simulink model "drive_closed_loop_system"  (R2023b)
settings: Solver=FixedStepDiscrete  StartTime=0.0  StopTime=0.1  FixedStep=Ts  RelTol=1e-3
model workspace (MATLAB code in the model file):
  | % Top-level execution parameter
  | % Placeholder value for structural closed-loop execution only.
  | 
  | Ts = 1e-6;      % top-level discrete step [s]
  | 
  | % Neutral default operating point for Phase-4 behavioural baseline
  | i_d_ref_default = 0;
  | i_q_ref_default = 10;
  | omega_e_default = 300;
  | 
  | % Current step response setup
  | i_q_ref_step_t = 0.02;
  | i_q_ref_step_init = i_q_ref_default;
  | i_q_ref_step_final = i_q_ref_default;
  | 
  | % Load disturbance setup
  | omega_e_step_t = 0.02;
  | omega_e_init = omega_e_default;
  | omega_e_step_final = omega_e_default;
undefined symbols (not defined in the file): DiscIntNeverNeededParam
libraries: sps_lib x1
settings Model: Creator=hwma  LastModifiedBy=hwma

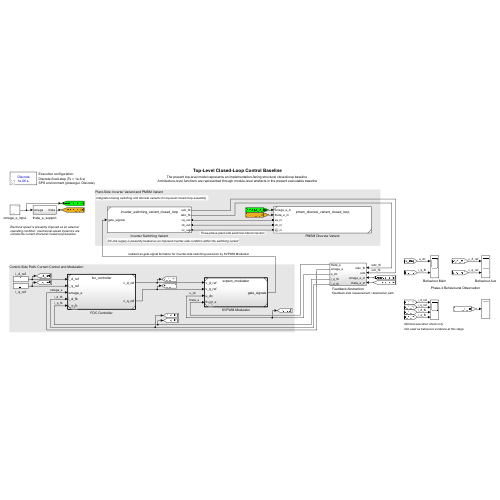
[thumbnail: Simulink's stored preview of the top-level diagram]
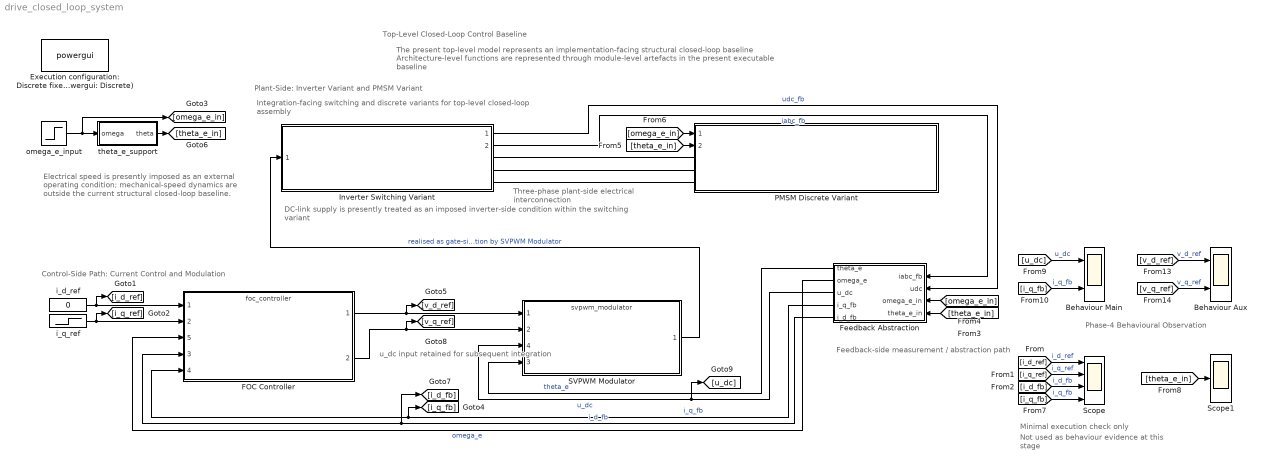
== system drive_closed_loop_system ==
  note: Phase-4 Behavioural Observation
  note: Minimal execution check only
  note: DC-link supply is presently treated as an imposed inverter-side condition within the switching variant
  note: Electrical speed is presently imposed as an external operating condition; mechanical-speed dynamics are outside the current structural closed-loop baseline.
  note: Three-phase plant-side electrical interconnection
  note: Feedback-side measurement / abstraction path
  note: Integration-facing switching and discrete variants for top-level closed-loop assembly
  note: Control-Side Path: Current Control and Modulation
  note: u_dc input retained for subsequent integration
  note: The present top-level model represents an implementation-facing structural closed-loop baseline
      | Architecture-level functions are represented through module-level artefacts in the present executable baseline
  note: Top-Level Closed-Loop Control Baseline
  note: Plant-Side: Inverter Variant and PMSM Variant
  note: Not used as behaviour evidence at this stage
  Behaviour Aux : Scope  NumInputPorts=2
  Behaviour Main : Scope  NumInputPorts=2
  Execution configuration: Discrete fixed-step (Ts = 1e-6 s) SPS environment (powergui: Discrete) : sps_lib/powergui  Priority=1  SimulationMode=Discrete  SampleTime=Ts  frequency=60  Iterations=50  frequencyindice=0  Pbase=100e6  ErrMax=1e-4  UnitsV=kV  UnitsW=MW  buscounter=0  FunctionMessages=off  echomessages=off  EnableUseOfTLC=off  CurrentSourceSwitches=off  DisableSnubberDevices=off  DisableRonSwitches=off  DisableVfSwitches=off  DisplayEquations=off  AutomaticDiscreteSolvers=off  SolverType=Tustin/Backward Euler (TBE)  Interpol=off  ExternalGateDelay=off  methode=off  Ts=100  x0status=blocks  SPID=on  SwTol=0  HookPort=off  NonlinearTolerance=1e-4  nMaxIteration=100  ContinueOnMaxIteration=off  RestoreLinks=warning  ResistiveCurrentMeasurement=off  Frange=[0:2:500]  Ylog=off  Xlog=on  ShowGrid=off  save=off  variable=ZData  structure=0  ZoomFFT=off  StartTime=0.0  cycles=1  DisplayStyle=1  fundamental=60  FreqAxis=off  MaxFrequency=1000  frequencyindicesteady=1  RmsSteady=1  display=off
  FOC Controller : ModelReference  ModelNameDialog=foc_controller.slx  SimulationMode=Normal  ModelReferenceVersion=1.26
      settings: PortSchema="{\"entries\":[{\"content\":{\"sides\":[{\"content\":{\"connectorIds\":[\"In1\",\"In2\",\"In5\",\"In3\",\"In4\"]},\"type\":\"ConnectorPlacement.EquallySpacedRectSide\",\"uuid\":\"ef112b4b-a133-4498-b633-78f8f1506d01\"},{\"content\":{\"connectorIds\":[\"Out1\",\"Out2\"],\"side\":\"RIGHT\"},\"type\":\"ConnectorPlacement.EquallySpacedRectSide\",\"uuid\":\"9847a18b-aaef-4243-aa5c-65f99a7910c1\"},{\"content\":{\"side\":\"TOP\"},\"type\":\"ConnectorPlacement.EquallySpacedRectSide\",\"uuid\":\"77b91c6a-a91c-4edb-91a8-4515c999bc11\"}]},\"type\":\"ConnectorPlacement.EquallySpacedConnector\",\"uuid\":\"240ede47-394a-4747-9d30-c9f3a7878d8f\"}],\"packageUris\":[\"http://schema.mathworks.com/mf0/Connector/R2020b\"],\"version\":\"1.0\"}"
  Feedback Abstraction : Subsystem
  Inverter Switching Variant : Subsystem  ReferencedSubsystem=inverter_switching_variant_closed_loop
  PMSM Discrete Variant : Subsystem  ReferencedSubsystem=pmsm_discrete_variant_closed_loop  Rs=0.05  Ld=2e-3  Lq=2e-3  lambda_f=0.1
  SVPWM Modulator : ModelReference  ModelNameDialog=svpwm_modulator.slx  SimulationMode=Normal  ModelReferenceVersion=1.34
      settings: PortSchema="{\"entries\":[{\"content\":{\"sides\":[{\"content\":{\"connectorIds\":[\"In1\",\"In2\",\"In4\",\"In3\"]},\"type\":\"ConnectorPlacement.EquallySpacedRectSide\",\"uuid\":\"0e0645a3-2a27-4c15-9a47-960d3777f31f\"},{\"content\":{\"connectorIds\":[\"Out1\"],\"side\":\"RIGHT\"},\"type\":\"ConnectorPlacement.EquallySpacedRectSide\",\"uuid\":\"17890dc1-ee5f-46a3-bfa4-af9c9726f2d2\"},{\"content\":{\"side\":\"TOP\"},\"type\":\"ConnectorPlacement.EquallySpacedRectSide\",\"uuid\":\"20a4fc6c-c015-4803-8581-584a4f0c357e\"}]},\"type\":\"ConnectorPlacement.EquallySpacedConnector\",\"uuid\":\"32cc6c3a-ba2d-4e41-b4c2-e07b22b54d61\"}],\"packageUris\":[\"http://schema.mathworks.com/mf0/Connector/R2020b\"],\"version\":\"1.0\"}"
  Scope : Scope  NumInputPorts=4
  Scope1 : Scope
  i_d_ref : Constant  Value=0  SampleTime=Ts
  i_q_ref : Step  Time=i_q_ref_step_t  Before=i_q_ref_step_init  After=i_q_ref_step_final  SampleTime=Ts
  omega_e_input : Step  Time=omega_e_step_t  Before=omega_e_init  After=omega_e_step_final  SampleTime=Ts
  theta_e_support : Subsystem
  wires:
  i_d_ref/1 -> FOC Controller/1, [i_d_ref]
  i_q_ref/1 -> [i_q_ref], FOC Controller/2
  FOC Controller/1 -> [v_d_ref], SVPWM Modulator/1
  FOC Controller/2 -> [v_q_ref], SVPWM Modulator/2
  SVPWM Modulator/1 -> Inverter Switching Variant/1  "realised as gate-signal formation for inverter-side switching execution by SVPWM Modulator"
  Inverter Switching Variant/1 -> Feedback Abstraction/2(udc)  "udc_fb"
  Inverter Switching Variant/2 -> Feedback Abstraction/1(iabc_fb)  "iabc_fb"
  Feedback Abstraction/5(i_d_fb) -> [i_d_fb], FOC Controller/3  "i_d_fb"
  Feedback Abstraction/4(i_q_fb) -> [i_q_fb], FOC Controller/4  "i_q_fb"
  Feedback Abstraction/3(u_dc) -> [u_dc], SVPWM Modulator/4  "u_dc"
  [omega_e_in] -> Feedback Abstraction/3(omega_e_in)
  omega_e_input/1 -> theta_e_support/1(omega), [omega_e_in]
  [theta_e_in] -> Feedback Abstraction/4(theta_e_in)
  [theta_e_in] -> PMSM Discrete Variant/2
  [omega_e_in] -> PMSM Discrete Variant/1
  Feedback Abstraction/1(theta_e) -> SVPWM Modulator/3  "theta_e"
  Feedback Abstraction/2(omega_e) -> FOC Controller/5  "omega_e"
  theta_e_support/1(theta) -> [theta_e_in]
  [i_d_ref] -> Scope/1  "i_d_ref"
  [i_q_ref] -> Scope/2  "i_q_ref"
  [i_d_fb] -> Scope/3  "i_d_fb"
  [i_q_fb] -> Scope/4  "i_q_fb"
  [theta_e_in] -> Scope1/1
  [u_dc] -> Behaviour Main/1  "u_dc"
  [i_q_fb] -> Behaviour Main/2  "i_q_fb"
  [v_q_ref] -> Behaviour Aux/2  "v_q_ref"
  [v_d_ref] -> Behaviour Aux/1  "v_d_ref"
  connections:
  Inverter Switching Variant/RConn1 -- PMSM Discrete Variant/LConn1
  Inverter Switching Variant/RConn2 -- PMSM Discrete Variant/LConn2
  Inverter Switching Variant/RConn3 -- PMSM Discrete Variant/LConn3

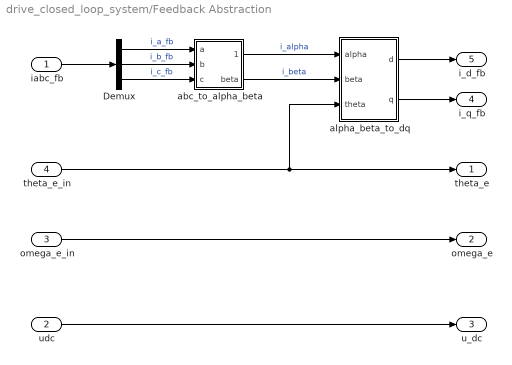
== system drive_closed_loop_system/Feedback Abstraction ==
  iabc_fb : Inport
  udc : Inport  Port=2
  omega_e_in : Inport  Port=3
  theta_e_in : Inport  Port=4
  Demux : Demux  Outputs=3
  abc_to_alpha_beta : Subsystem
  alpha_beta_to_dq : Subsystem
  theta_e : Outport
  omega_e : Outport  Port=2
  u_dc : Outport  Port=3
  i_q_fb : Outport  Port=4
  i_d_fb : Outport  Port=5
  wires:
  iabc_fb/1 -> Demux/1
  Demux/3 -> abc_to_alpha_beta/3(c)  "i_c_fb"
  Demux/2 -> abc_to_alpha_beta/2(b)  "i_b_fb"
  Demux/1 -> abc_to_alpha_beta/1(a)  "i_a_fb"
  abc_to_alpha_beta/2(beta) -> alpha_beta_to_dq/2(beta)  "i_beta"
  abc_to_alpha_beta/1(alpha) -> alpha_beta_to_dq/1(alpha)  "i_alpha"
  alpha_beta_to_dq/1(d) -> i_d_fb/1
  alpha_beta_to_dq/2(q) -> i_q_fb/1
  udc/1 -> u_dc/1
  omega_e_in/1 -> omega_e/1
  theta_e_in/1 -> alpha_beta_to_dq/3(theta), theta_e/1

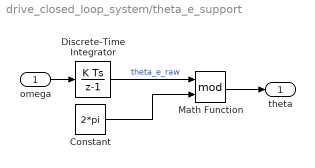
== system drive_closed_loop_system/theta_e_support ==
  omega : Inport
  Constant : Constant  Value=2*pi
  Discrete-Time Integrator : DiscreteIntegrator  SampleTime=Ts  ICPrevOutput=DiscIntNeverNeededParam  ICPrevScaledInput=DiscIntNeverNeededParam
  Math Function : Math  Operator=mod
  theta : Outport
  wires:
  Constant/1 -> Math Function/2
  Math Function/1 -> theta/1
  omega/1 -> Discrete-Time Integrator/1
  Discrete-Time Integrator/1 -> Math Function/1  "theta_e_raw"

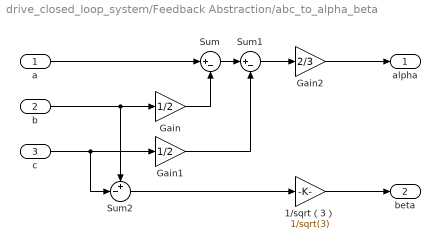
== system drive_closed_loop_system/Feedback Abstraction/abc_to_alpha_beta ==
  a : Inport
  b : Inport  Port=2
  c : Inport  Port=3
  1/sqrt（3） : Gain  Gain=1/sqrt(3)
  Gain : Gain  Gain=1/2
  Gain1 : Gain  Gain=1/2
  Gain2 : Gain  Gain=2/3
  Sum : Sum  Inputs=|+-
  Sum1 : Sum  Inputs=|+-
  Sum2 : Sum  Inputs=+-|
  alpha : Outport
  beta : Outport  Port=2
  wires:
  a/1 -> Sum/1
  b/1 -> Sum2/1, Gain/1
  c/1 -> Sum2/2, Gain1/1
  Gain/1 -> Sum/2
  Sum/1 -> Sum1/1
  Gain1/1 -> Sum1/2
  Sum1/1 -> Gain2/1
  Gain2/1 -> alpha/1
  Sum2/1 -> 1/sqrt（3）/1
  1/sqrt（3）/1 -> beta/1

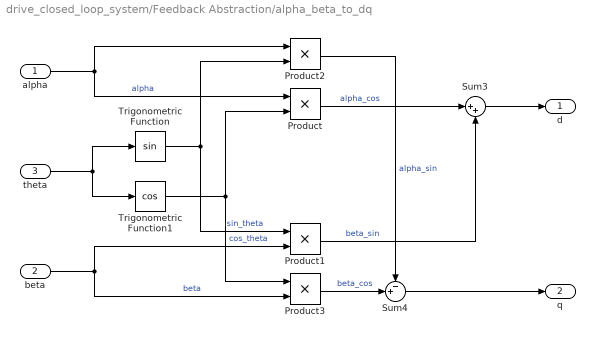
== system drive_closed_loop_system/Feedback Abstraction/alpha_beta_to_dq ==
  alpha : Inport
  beta : Inport  Port=2
  theta : Inport  Port=3
  Product{,1..3} (4 alike) : Product
  Sum3 : Sum  Inputs=|++
  Sum4 : Sum  Inputs=-+|
  Trigonometric Function : Trigonometry
  Trigonometric Function1 : Trigonometry  Operator=cos
  d : Outport
  q : Outport  Port=2
  wires:
  theta/1 -> Trigonometric Function1/1, Trigonometric Function/1
  alpha/1 -> Product2/1, Product/1  "alpha"
  Trigonometric Function1/1 -> Product3/1, Product/2  "cos_theta"
  beta/1 -> Product3/2, Product1/2  "beta"
  Trigonometric Function/1 -> Product2/2, Product1/1  "sin_theta"
  Product/1 -> Sum3/1  "alpha_cos"
  Product1/1 -> Sum3/2  "beta_sin"
  Sum3/1 -> d/1
  Product3/1 -> Sum4/2  "beta_cos"
  Product2/1 -> Sum4/1  "alpha_sin"
  Sum4/1 -> q/1
